simulink model "robotref"  (Simulink 6.3)
settings: Solver=ode45  StartTime=0.0  StopTime=10.0  RelTol=1e-3
settings Model: Creator=mbharadw  LastModifiedBy=mbharadw  ExtModeTrigMode=oneshot  ExtModeArmWhenConnect=off  StrictBusMsg=None
settings DataIOCC: LimitDataPoints=off
settings OptimizationCC: BlockReduction=off  BooleanDataType=off
settings DebuggingCC: SolverPrmCheckMsg=none
settings HardwareCC: TargetUnknown=on

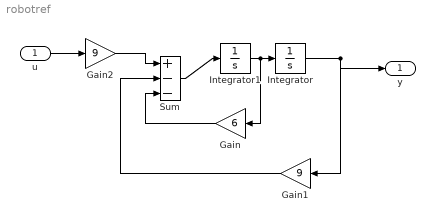
== system robotref ==
  u : Inport
  Gain : Gain  Orientation=left  Gain=6  SaturateOnIntegerOverflow=on
  Gain1 : Gain  Orientation=left  Gain=9  SaturateOnIntegerOverflow=on
  Gain2 : Gain  Gain=9  SaturateOnIntegerOverflow=on
  Integrator : Integrator
  Integrator1 : Integrator
  Sum : Sum  Inputs=+--  SaturateOnIntegerOverflow=on  InputSameDT=on
  y : Outport
  wires:
  Integrator/1 -> y/1, Gain1/1
  Sum/1 -> Integrator1/1
  Gain1/1 -> Sum/2
  Integrator1/1 -> Integrator/1, Gain/1
  Gain/1 -> Sum/3
  Gain2/1 -> Sum/1
  u/1 -> Gain2/1
